simulink model "double_transmission"  (R2015a)
settings: Solver=ode45  StartTime=0.0  StopTime=10.0  RelTol=1e-3
libraries: powerlib x15
settings Model: Creator=Sanchit  LastModifiedBy=Sanchit

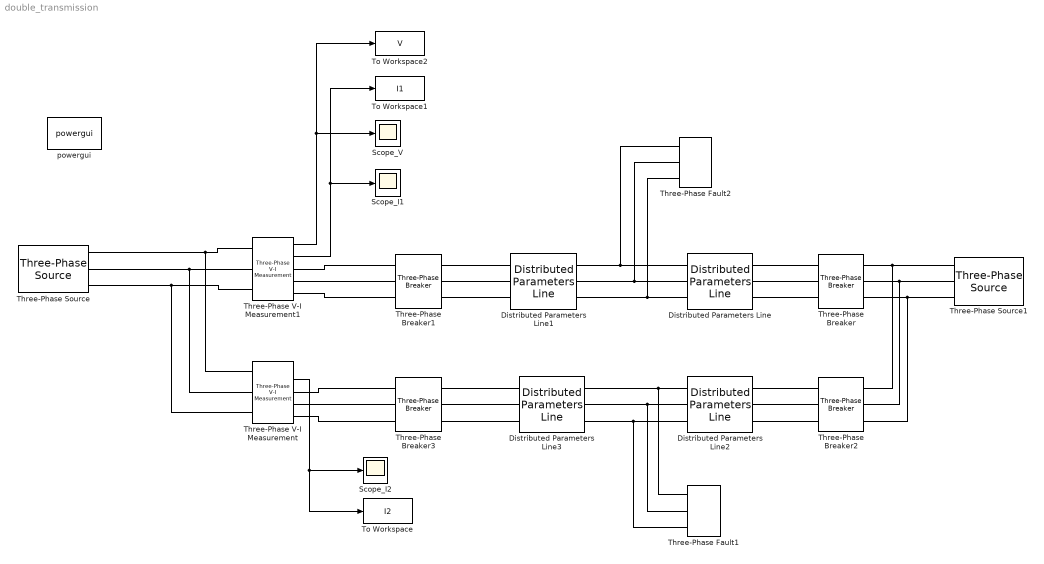
== system double_transmission ==
  Distributed Parameters Line : powerlib/Elements/Distributed Parameters Line  Phases=3  Frequency=60  Resistance=[0.01273 0.3864]  Inductance="[0.9337e-3  4.1264e-3]"  Capacitance=[12.74e-9 7.751e-9]  Length=100  x1=[0 0 0 0; 0.0001244 0 0 0; 0.0002488 0 0 0; 0.0003733 0 0 0; 0.0004977 0 0 0; 0.0006221 0 0 0]  x2=[0 0 0 0; 0.0001244 0 0 0; 0.0002488 0 0 0; 0.0003733 0 0 0; 0.0004977 0 0 0; 0.0006221 0 0 0]  x3=[0 0 0 0; 0.0001244 0 0 0; 0.0002488 0 0 0; 0.0003733 0 0 0; 0.0004977 0 0 0; 0.0006221 0 0 0]  x4=[0 0 0 0; 0.0001244 0 0 0; 0.0002488 0 0 0; 0.0003733 0 0 0; 0.0004977 0 0 0; 0.0006221 0 0 0]  x5=0  V1=[8.175e-11 457 457;314.2 314.2 314.2;1.319 -1.151 -2.722]  V2=[8.761e-11 455.2 455.2;314.2 314.2 314.2;1.353 -1.151 -2.722]  I1=[1.472e-13 1.683 1.683;314.2 314.2 314.2;1.017 -1.169 -2.74]  I2=[8.74e-14 1.682 1.682;314.2 314.2 314.2;1.639 -1.242 -2.812]  nHarmo=1  Measurements=None
  Distributed Parameters Line1 : powerlib/Elements/Distributed Parameters Line  Phases=3  Frequency=60  Resistance=[0.01273 0.3864]  Inductance="[0.9337e-3  4.1264e-3]"  Capacitance=[12.74e-9 7.751e-9]  Length=Lf  x1=[0 0 0 0; 0.0001244 0 0 0; 0.0002488 0 0 0; 0.0003733 0 0 0; 0.0004977 0 0 0; 0.0006221 0 0 0]  x2=[0 0 0 0; 0.0001244 0 0 0; 0.0002488 0 0 0; 0.0003733 0 0 0; 0.0004977 0 0 0; 0.0006221 0 0 0]  x3=[0 0 0 0; 0.0001244 0 0 0; 0.0002488 0 0 0; 0.0003733 0 0 0; 0.0004977 0 0 0; 0.0006221 0 0 0]  x4=[0 0 0 0; 0.0001244 0 0 0; 0.0002488 0 0 0; 0.0003733 0 0 0; 0.0004977 0 0 0; 0.0006221 0 0 0]  x5=0  V1=[7.695e-11 455.2 455.2;314.2 314.2 314.2;1.36 -1.115 -2.686]  V2=[8.175e-11 457 457;314.2 314.2 314.2;1.377 -1.115 -2.686]  I1=[1.402e-13 1.684 1.684;314.2 314.2 314.2;0.9977 -1.206 -2.777]  I2=[8.974e-14 1.685 1.685;314.2 314.2 314.2;1.835 -1.097 -2.668]  nHarmo=1  Measurements=None
  Distributed Parameters Line2 : powerlib/Elements/Distributed Parameters Line  Phases=3  Frequency=60  Resistance=[0.01273 0.3864]  Inductance="[0.9337e-3  4.1264e-3]"  Capacitance=[12.74e-9 7.751e-9]  Length=100  x1=[0 0 0 0; 0.0001244 0 0 0; 0.0002488 0 0 0; 0.0003733 0 0 0; 0.0004977 0 0 0; 0.0006221 0 0 0]  x2=[0 0 0 0; 0.0001244 0 0 0; 0.0002488 0 0 0; 0.0003733 0 0 0; 0.0004977 0 0 0; 0.0006221 0 0 0]  x3=[0 0 0 0; 0.0001244 0 0 0; 0.0002488 0 0 0; 0.0003733 0 0 0; 0.0004977 0 0 0; 0.0006221 0 0 0]  x4=[0 0 0 0; 0.0001244 0 0 0; 0.0002488 0 0 0; 0.0003733 0 0 0; 0.0004977 0 0 0; 0.0006221 0 0 0]  x5=0  V1=[1.564e-09 457 457;314.2 314.2 314.2;-0.8833 -1.151 -2.722]  V2=[1.573e-09 455.2 455.2;314.2 314.2 314.2;-0.873 -1.151 -2.722]  I1=[2.202e-12 1.683 1.683;314.2 314.2 314.2;-0.9807 -1.169 -2.74]  I2=[1.947e-12 1.682 1.682;314.2 314.2 314.2;-0.955 -1.242 -2.812]  nHarmo=1  Measurements=None
  Distributed Parameters Line3 : powerlib/Elements/Distributed Parameters Line  Phases=3  Frequency=60  Resistance=[0.01273 0.3864]  Inductance="[0.9337e-3  4.1264e-3]"  Capacitance=[12.74e-9 7.751e-9]  Length=Lf  x1=[0 0 0 0; 0.0001244 0 0 0; 0.0002488 0 0 0; 0.0003733 0 0 0; 0.0004977 0 0 0; 0.0006221 0 0 0]  x2=[0 0 0 0; 0.0001244 0 0 0; 0.0002488 0 0 0; 0.0003733 0 0 0; 0.0004977 0 0 0; 0.0006221 0 0 0]  x3=[0 0 0 0; 0.0001244 0 0 0; 0.0002488 0 0 0; 0.0003733 0 0 0; 0.0004977 0 0 0; 0.0006221 0 0 0]  x4=[0 0 0 0; 0.0001244 0 0 0; 0.0002488 0 0 0; 0.0003733 0 0 0; 0.0004977 0 0 0; 0.0006221 0 0 0]  x5=0  V1=[1.53e-09 455.2 455.2;314.2 314.2 314.2;-0.8263 -1.115 -2.686]  V2=[1.564e-09 457 457;314.2 314.2 314.2;-0.8247 -1.115 -2.686]  I1=[2.221e-12 1.684 1.684;314.2 314.2 314.2;-1.036 -1.206 -2.777]  I2=[1.969e-12 1.685 1.685;314.2 314.2 314.2;-0.7158 -1.097 -2.668]  nHarmo=1  Measurements=None
  Scope_I1 : Scope
      settings: SaveName=ScopeData2
  Scope_I2 : Scope
  Scope_V : Scope
      settings: SaveName=ScopeData3
  Three-Phase V-I Measurement : powerlib/Measurements/Three-Phase V-I Measurement  VoltageMeasurement=phase-to-ground  SetLabelV=off  LabelV=Vabc  Vpu=off  VpuLL=off  CurrentMeasurement=yes  SetLabelI=off  LabelI=Iabc  Ipu=off  Pbase=100e6  Vbase=500e3  OutputType=Complex  PhasorSimulation=off  PSBequivalent=0
  Three-Phase V-I Measurement1 : powerlib/Measurements/Three-Phase V-I Measurement  VoltageMeasurement=phase-to-ground  SetLabelV=off  LabelV=Vabc  Vpu=off  VpuLL=off  CurrentMeasurement=yes  SetLabelI=off  LabelI=Iabc  Ipu=off  Pbase=100e6  Vbase=500e3  OutputType=Complex  PhasorSimulation=off  PSBequivalent=0
  Three-Phase Breaker{,1..3} (4 alike) : powerlib/Elements/Three-Phase Breaker  InitialState=open  SwitchA=on  SwitchB=on  SwitchC=on  SwitchTimes="[1/60  5/60]"  External=off  BreakerResistance=0.01  SnubberResistance=1e6  SnubberCapacitance=inf  Measurements=None
  Three-Phase Fault1 : powerlib/Elements/Three-Phase Fault  InitialStates=0  FaultA=on  FaultB=on  FaultC=on  GroundFault=on  SwitchTimes="[1/60  5/60]"  External=off  SwitchStatus=NaN  FaultResistance=Rf  GroundResistance=0.01  SnubberResistance=1e6  SnubberCapacitance=inf  Measurements=None
  Three-Phase Fault2 : powerlib/Elements/Three-Phase Fault  InitialStates=0  FaultA=on  FaultB=on  FaultC=on  GroundFault=on  SwitchTimes="[1/60  5/60]"  External=off  SwitchStatus=NaN  FaultResistance=Rf  GroundResistance=0.01  SnubberResistance=1e6  SnubberCapacitance=inf  Measurements=None
  Three-Phase Source : powerlib/Electrical Sources/Three-Phase Source  Voltage=152.54e3  PhaseAngle=0  Frequency=50  InternalConnection=Yg  SpecifyImpedance=on  Resistance=0.8929  Inductance=16.58e-3  ShortCircuitLevel=100e6  BaseVoltage=25e3  XRratio=7  BusType=swing  Pref=0  Qref=0  Qmin=-inf  Qmax=inf
  Three-Phase Source1 : powerlib/Electrical Sources/Three-Phase Source  Voltage=152.54e3  PhaseAngle=0  Frequency=50  InternalConnection=Yg  SpecifyImpedance=on  Resistance=0.8929  Inductance=16.58e-3  ShortCircuitLevel=100e6  BaseVoltage=25e3  XRratio=7  BusType=swing  Pref=0  Qref=0  Qmin=-inf  Qmax=inf
  To Workspace : ToWorkspace  VariableName=I2  SaveFormat=Timeseries  SampleTime=-1
  To Workspace1 : ToWorkspace  VariableName=I1  SaveFormat=Timeseries  SampleTime=-1
  To Workspace2 : ToWorkspace  VariableName=V  SaveFormat=Timeseries  SampleTime=-1
  powergui : powerlib/powergui  Priority=1  SimulationMode=Continuous  SolverType=Tustin/Backward Euler (TBE)  SampleTime=50e-6  frequency=60  SPID=off  DisableSnubberDevices=off  DisableRonSwitches=off  DisableVfSwitches=off  SwTol=0  DisplayEquations=off  Interpol=off  methode=off  Ts=100  FunctionMessages=off  echomessages=off  HookPort=off  EnableUseOfTLC=off  x0status=blocks  frequencyindice=50  Pbase=100e6  ErrMax=1e-4  Iterations=50  UnitsV=kV  UnitsW=MW  buscounter=0  RestoreLinks=warning  ResistiveCurrentMeasurement=off  Frange=[0:2:500]  Ylog=off  Xlog=on  ShowGrid=off  save=off  variable=ZData  structure=0  ZoomFFT=off  StartTime=0.0  cycles=1  DisplayStyle=1  fundamental=60  FreqAxis=off  MaxFrequency=1000  frequencyindicesteady=1  RmsSteady=1  display=off
  wires:
  Three-Phase V-I Measurement1/1 -> To Workspace2/1, Scope_V/1
  Three-Phase V-I Measurement1/2 -> To Workspace1/1, Scope_I1/1
  Three-Phase V-I Measurement/2 -> To Workspace/1, Scope_I2/1
  connections:
  Three-Phase Breaker1/RConn1 -- Distributed Parameters Line1/LConn1
  Three-Phase Breaker1/RConn2 -- Distributed Parameters Line1/LConn2
  Three-Phase Breaker1/RConn3 -- Distributed Parameters Line1/LConn3
  Three-Phase Breaker3/RConn1 -- Distributed Parameters Line3/LConn1
  Three-Phase Breaker3/RConn2 -- Distributed Parameters Line3/LConn2
  Three-Phase Breaker3/RConn3 -- Distributed Parameters Line3/LConn3
  Distributed Parameters Line2/RConn1 -- Three-Phase Breaker2/LConn1
  Distributed Parameters Line2/RConn2 -- Three-Phase Breaker2/LConn2
  Distributed Parameters Line2/RConn3 -- Three-Phase Breaker2/LConn3
  Distributed Parameters Line/RConn3 -- Three-Phase Breaker/LConn3
  Distributed Parameters Line/RConn2 -- Three-Phase Breaker/LConn2
  Distributed Parameters Line/RConn1 -- Three-Phase Breaker/LConn1
  Three-Phase Source/RConn1 -- Three-Phase V-I Measurement/LConn1 -- Three-Phase V-I Measurement1/LConn1
  Three-Phase Breaker/RConn1 -- Three-Phase Breaker2/RConn1 -- Three-Phase Source1/RConn1
  Three-Phase Source/RConn2 -- Three-Phase V-I Measurement/LConn2 -- Three-Phase V-I Measurement1/LConn2
  Three-Phase Source/RConn3 -- Three-Phase V-I Measurement/LConn3 -- Three-Phase V-I Measurement1/LConn3
  Three-Phase Breaker/RConn2 -- Three-Phase Breaker2/RConn2 -- Three-Phase Source1/RConn2
  Three-Phase Breaker/RConn3 -- Three-Phase Breaker2/RConn3 -- Three-Phase Source1/RConn3
  Three-Phase V-I Measurement1/RConn2 -- Three-Phase Breaker1/LConn2
  Three-Phase V-I Measurement1/RConn3 -- Three-Phase Breaker1/LConn3
  Three-Phase V-I Measurement1/RConn1 -- Three-Phase Breaker1/LConn1
  Distributed Parameters Line1/RConn1 -- Three-Phase Fault2/LConn1 -- Distributed Parameters Line/LConn1
  Distributed Parameters Line1/RConn2 -- Three-Phase Fault2/LConn2 -- Distributed Parameters Line/LConn2
  Distributed Parameters Line1/RConn3 -- Three-Phase Fault2/LConn3 -- Distributed Parameters Line/LConn3
  Distributed Parameters Line3/RConn1 -- Three-Phase Fault1/LConn1 -- Distributed Parameters Line2/LConn1
  Distributed Parameters Line3/RConn2 -- Three-Phase Fault1/LConn2 -- Distributed Parameters Line2/LConn2
  Distributed Parameters Line3/RConn3 -- Three-Phase Fault1/LConn3 -- Distributed Parameters Line2/LConn3
  Three-Phase V-I Measurement/RConn2 -- Three-Phase Breaker3/LConn2
  Three-Phase V-I Measurement/RConn1 -- Three-Phase Breaker3/LConn1
  Three-Phase V-I Measurement/RConn3 -- Three-Phase Breaker3/LConn3
